simulink model "ModerForV"  (R2016a)
settings: Solver=ode3  StartTime=0.0  StopTime=0.0050  FixedStep=1e-7  MaxStep=1e-6  RelTol=1e-3
libraries: simulink x1
settings Model: Creator=pankx  LastModifiedBy=WangChao
settings DataIOCC: LimitDataPoints=on  SaveFormat=Array  SignalLoggingSaveFormat=ModelDataLogs  InspectSignalLogs=on
settings OptimizationCC: InitFltsAndDblsToZero=on
settings DebuggingCC: SaveWithParameterizedLinksMsg=none  UnderspecifiedInitializationDetection=Classic  MergeDetectMultiDrivingBlocksExec=none  SignalResolutionControl=TryResolveAllWithWarning  SolverPrmCheckMsg=warning  MultiTaskDSMMsg=warning  MultiTaskCondExecSysMsg=none  FcnCallInpInsideContextMsg=UseLocalSettings  StateNameClashWarn=warning
settings HardwareCC: ProdBitPerPointer=32  ProdLargestAtomicFloat=None  ProdIntDivRoundTo=Undefined  ProdEndianess=Unspecified  ProdWordSize=32  ProdHWDeviceType=32-bit Generic
settings ModelReferenceCC: PropagateSignalLabelsOutOfModel=off
settings GRTTargetCC: TargetFcnLib=ansi_tfl_tmw.mat  CombineOutputUpdateFcns=off  GRTInterface=on
settings ConfigComp: CovModelRefEnable=Off

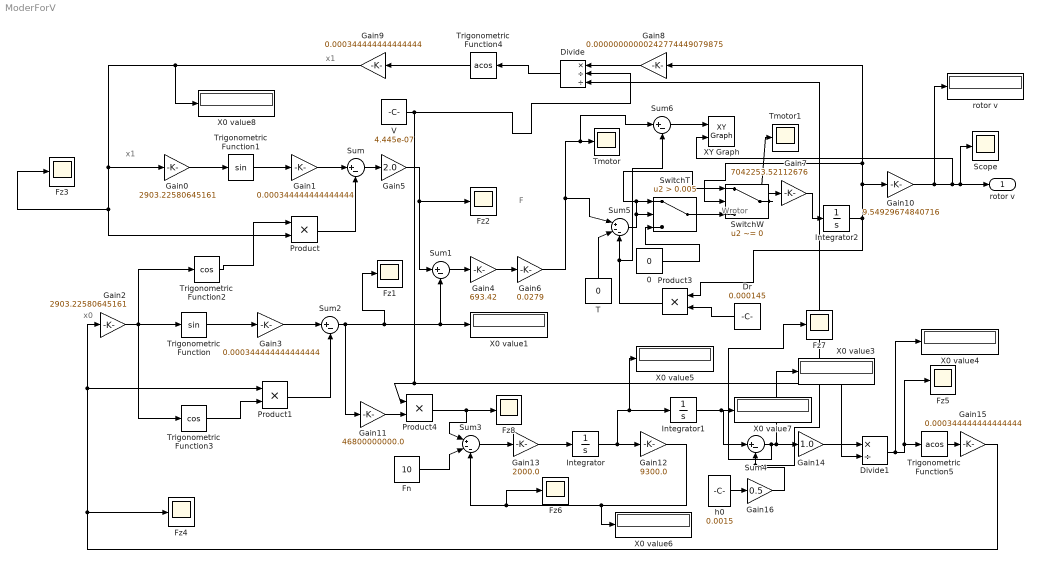
== system ModerForV ==
  note: x0
  note: x1
  note: F
  note: Wrotor
  note: x1
   X0 value{1,3..8} (7 alike) : Display
  0 : Constant  Value=0
  Divide : Product  Inputs=*//
  Divide1 : Product  Inputs=*/
  Dr : Constant  Value=0.000145
  Fn : Constant  Value=10
  Fz{1..8} (8 alike) : Scope
  Gain0 : Gain  Gain=2903.22580645161
  Gain{1,3,9,15} (4 alike) : Gain  Gain=0.000344444444444444
  Gain10 : Gain  Gain=9.54929674840716
  Gain11 : Gain  Gain=46800000000.0
  Gain12 : Gain  Gain=9300.0
  Gain13 : Gain  Gain=2000.0
  Gain14 : Gain  Gain=1.0
  Gain16 : Gain  Gain=0.5
  Gain2 : Gain  Gain=2903.22580645161
  Gain4 : Gain  Gain=693.42
  Gain5 : Gain  Gain=2.0
  Gain6 : Gain  Gain=0.0279
  Gain7 : Gain  Gain=7042253.52112676
  Gain8 : Gain  Gain=0.00000000000242774449079875
  Integrator : Integrator
  Integrator1 : Integrator  InitialCondition=0.00075
  Integrator2 : Integrator
  Product{,1,3..4} (4 alike) : Product  RndMeth=Zero
  Scope : Scope
  Sum{,1..2,4,6} (5 alike) : Sum  Inputs=|+-
  Sum3 : Sum  Inputs=|+--
  Sum5 : Sum  Inputs=|+--
  SwitchT : Switch  Criteria=u2 > Threshold  Threshold=0.005
  SwitchW : Switch  Criteria=u2 ~= 0
  T : Constant  Value=0
  Tmotor : Scope
  Tmotor1 : Scope
  Trigonometric Function : Trigonometry
  Trigonometric Function1 : Trigonometry
  Trigonometric Function2 : Trigonometry  Operator=cos
  Trigonometric Function3 : Trigonometry  Operator=cos
  Trigonometric Function4 : Trigonometry  Operator=acos
  Trigonometric Function5 : Trigonometry  Operator=acos
  V : Constant  Value=4.445e-07
  XY Graph : simulink/Sinks/XY Graph  xmin=0  xmax=0.03  ymin=0  ymax=1000  st=-1
  h0 : Constant  Value=0.0015
  rotor v : Display
  "rotor v " : Outport
  wires:
  Gain0/1 -> Trigonometric Function1/1
  Trigonometric Function1/1 -> Gain1/1
  Gain1/1 -> Sum/1
  Sum/1 -> Gain5/1
  Trigonometric Function2/1 -> Product/1
  Gain5/1 -> Fz2/1, Sum1/1
  Trigonometric Function/1 -> Gain3/1
  Gain3/1 -> Sum2/1
  Trigonometric Function3/1 -> Product1/2
  Product1/1 -> Sum2/2
  Fn/1 -> Sum3/2
  Gain12/1 -> " X0 value6"/1, Fz6/1, Sum3/3
  Sum2/1 -> Fz1/1, " X0 value1"/1, Sum1/2, Gain11/1
  Gain2/1 -> Trigonometric Function2/1, Trigonometric Function3/1, Trigonometric Function/1
  Sum3/1 -> Gain13/1
  Gain13/1 -> Integrator/1
  Integrator/1 -> " X0 value5"/1, Integrator1/1, Gain12/1
  Trigonometric Function4/1 -> Gain9/1
  Product/1 -> Sum/2
  Sum1/1 -> Gain4/1
  Gain4/1 -> Gain6/1
  Sum5/1 -> SwitchW/1, SwitchT/1, SwitchT/2
  Gain7/1 -> Integrator2/1
  Gain10/1 -> rotor v/1, XY Graph/2, "rotor v "/1, Scope/1
  T/1 -> Sum5/2
  Trigonometric Function5/1 -> Gain15/1
  Integrator2/1 -> Product3/1, SwitchW/2, Gain8/1, Gain10/1
  Dr/1 -> Product3/2
  Product3/1 -> Sum6/2, Sum5/3
  Gain8/1 -> Divide/1
  Divide/1 -> Trigonometric Function4/1
  V/1 -> Divide/2, Product4/1, Divide1/2
  Gain11/1 -> Product4/2
  Product4/1 -> Sum3/1, Fz8/1
  h0/1 -> Gain16/1
  Gain16/1 -> Sum4/2, Divide/3
  Sum4/1 -> Fz7/1, " X0 value3"/1, Gain14/1
  Gain14/1 -> Divide1/1
  Divide1/1 -> " X0 value4"/1, Fz5/1, Trigonometric Function5/1
  Integrator1/1 -> " X0 value7"/1, Sum4/1
  Gain9/1 -> " X0 value8"/1, Fz3/1, Product/2, Gain0/1
  0/1 -> SwitchT/3
  SwitchT/1 -> SwitchW/3
  Gain6/1 -> Sum5/1, Sum6/1, Tmotor/1
  SwitchW/1 -> Gain7/1, Tmotor1/1
  Sum6/1 -> XY Graph/1
  Gain15/1 -> Product1/1, Gain2/1, Fz4/1
